simulink model "GA_tracking_sim"  (R2024a)
settings: Solver=FixedStepAuto  StartTime=0.0  StopTime=100  FixedStep=1e-3  RelTol=1e-3
InitFcn:
  | close;
  | % % z
  | k_p_z = -9.64;
  | k_i_z = -5.55;
  | k_d_z = -7.46;
  | k_a_z = 1.37;
  | %
  | % % psi
  | k_p_psi = 5.84;
  | k_d_psi = .836;
  | %
  | % % phi
  | k_p_phi = 2.33;
  | k_d_phi = 0.756;
  | %
  | % % tt
  | k_p_tt = 1;
  | k_d_tt = .302;
StopFcn:
  | % plot3(x,y,-z,['b','-'],x_g,y_g,z_g,['r','--'],'LineWidth',1.25);
  | % xlabel('x');
  | % ylabel('y');
  | % zlabel('z');
  | % grid on;
undefined symbols (not defined in the file or in its folder): k_a_phi, k_a_psi, k_a_tt, k_a_x, k_a_y, k_d_x, k_d_y, k_i_phi, k_i_psi, k_i_tt, k_i_x, k_i_y, k_p_x, k_p_y
libraries: simulink x6
settings Model: Creator=luand  LastModifiedBy=luand
settings DataIOCC: ReturnWorkspaceOutputs=off

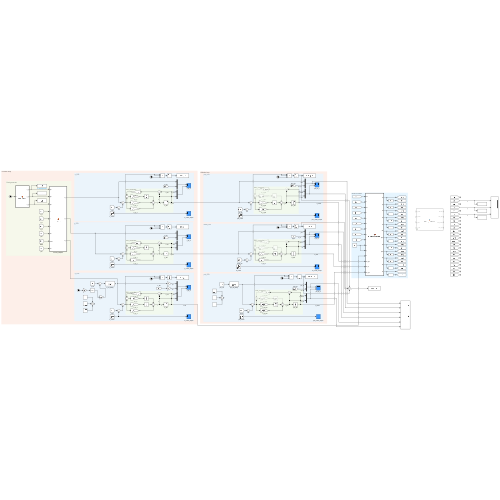
[thumbnail: Simulink's stored preview of the top-level diagram]
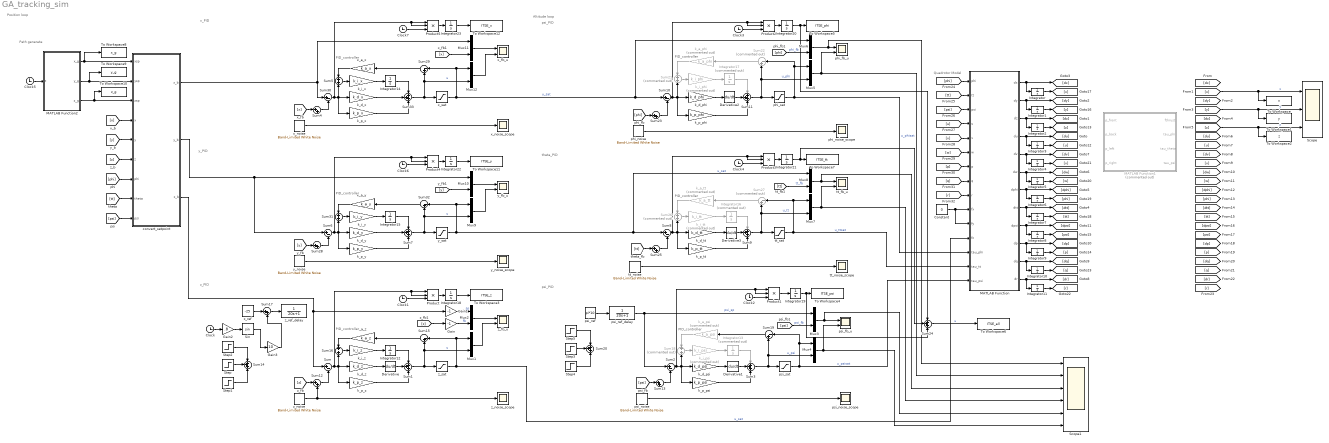
== system GA_tracking_sim ==
  note: Path generate
  note: Altitude loop
  note: z_PID
  note: PID_controller
  note: PID_controller
  note: psi_PID
  note: Quadrotor Model
  note: PID_controller
  note: PID_controller
  note: PID_controller
  note: PID_controller
  note: theta_PID
  note: psi_PID
  note: Position loop
  note: y_PID
  note: x_PID
  Clock{,1..7} (8 alike) : Clock
  Constant : Constant  Value=0
  Derivative{,1..3} (4 alike) : Derivative
  Gain : Gain  Gain=-1
  Gain1 : Gain  Gain=-1
  Gain2 : Gain  Gain=.8
  Gain3 : Gain  Gain=10
  Integrator : Integrator  UpperSaturationLimit=1000  LowerSaturationLimit=-1000
  Integrator1 : Integrator  UpperSaturationLimit=1000  LowerSaturationLimit=-1000
  Integrator{8..11} (4 alike) : Integrator  LimitOutput=on  UpperSaturationLimit=100  LowerSaturationLimit=-100
  Integrator12 : Integrator  UpperSaturationLimit=1000  LowerSaturationLimit=-1000
  Integrator13 : Integrator  Commented=on  LimitOutput=on  UpperSaturationLimit=1000  LowerSaturationLimit=-1000
  Integrator14 : Integrator
  Integrator15 : Integrator
  Integrator16 : Integrator  Commented=on
  Integrator17 : Integrator  Commented=on  LimitOutput=on  UpperSaturationLimit=1000  LowerSaturationLimit=-1000
  Integrator18 : Integrator  UpperSaturationLimit=100000  LowerSaturationLimit=-100000
  Integrator{19..23} (5 alike) : Integrator  LimitOutput=on  UpperSaturationLimit=100000  LowerSaturationLimit=-100000
  Integrator2 : Integrator  UpperSaturationLimit=0  LowerSaturationLimit=-1000
  Integrator3 : Integrator  LimitOutput=on  UpperSaturationLimit=10000  LowerSaturationLimit=-10000
  Integrator4 : Integrator  LimitOutput=on  UpperSaturationLimit=10000  LowerSaturationLimit=-10000
  Integrator5 : Integrator  LimitOutput=on  UpperSaturationLimit=10000  LowerSaturationLimit=-10000
  Integrator6 : Integrator  LimitOutput=on  UpperSaturationLimit=1000  LowerSaturationLimit=-1000
  Integrator7 : Integrator  LimitOutput=on  UpperSaturationLimit=1000  LowerSaturationLimit=-1000
  MATLAB Function : MATLAB Function  TreatAsAtomicUnit=on
  MATLAB Function1 : MATLAB Function  Commented=on  TreatAsAtomicUnit=on
  MATLAB Function2 : MATLAB Function  TreatAsAtomicUnit=on
  Mux{1..12} (12 alike) : Mux  Inputs=2
  Product{,1..5} (6 alike) : Product  Inputs=3
  Scope : Scope  NumInputPorts=3
  Scope1 : Scope  NumInputPorts=6
  Sin : Trigonometry
  Step : Step  Time=25  After=-20  SampleTime=0
  Step1 : Step  Time=40  After=15  SampleTime=0
  Step2 : Step  Time=10  After=-5  SampleTime=0
  Step3 : Step  Time=8  After=-6.28  SampleTime=0
  Step4 : Step  Time=17  After=6.28  SampleTime=0
  Step5 : Step  After=3.14  SampleTime=0
  Sum{,2,6,8,10,30} (6 alike) : Sum  Inputs=|+-
  Sum{1,3,7,9,11,14,20,24,33} (9 alike) : Sum  Inputs=+++
  Sum{4,12..13,17,23,25,28} (7 alike) : Sum  Inputs=|++
  Sum{15,19,29,32} (4 alike) : Sum  Inputs=|-+
  Sum16 : Sum  Inputs=+|+
  Sum18 : Sum  Commented=on  Inputs=+|+
  Sum21 : Sum  Commented=on  Inputs=+|+
  Sum22 : Sum  Commented=on  Inputs=|-+
  Sum26 : Sum  Commented=on  Inputs=+|+
  Sum27 : Sum  Commented=on  Inputs=|-+
  Sum31 : Sum  Inputs=+|+
  Sum5 : Sum  Inputs=+|+
  To Workspace : ToWorkspace  VariableName=x  SampleTime=-1
      settings: Save2DSignal=2-D array (concatenate along first dimension)
  To Workspace1 : ToWorkspace  VariableName=y  SampleTime=-1
      settings: Save2DSignal=2-D array (concatenate along first dimension)
  To Workspace10 : ToWorkspace  VariableName=z_g  SampleTime=-1
      settings: Save2DSignal=2-D array (concatenate along first dimension)
  To Workspace11 : ToWorkspace  VariableName=ITSE_y  SampleTime=-1
  To Workspace12 : ToWorkspace  VariableName=ITSE_x  SampleTime=-1
  To Workspace2 : ToWorkspace  VariableName=z  SampleTime=-1
      settings: Save2DSignal=2-D array (concatenate along first dimension)
  To Workspace3 : ToWorkspace  VariableName=ITSE_z  SampleTime=-1
  To Workspace4 : ToWorkspace  VariableName=ITSE_psi  SampleTime=-1
  To Workspace5 : ToWorkspace  VariableName=ITSE_phi  SampleTime=-1
  To Workspace6 : ToWorkspace  VariableName=ITSE_all  SampleTime=-1
  To Workspace7 : ToWorkspace  VariableName=ITSE_tt  SampleTime=-1
  To Workspace8 : ToWorkspace  VariableName=x_g  SampleTime=-1
      settings: Save2DSignal=2-D array (concatenate along first dimension)
  To Workspace9 : ToWorkspace  VariableName=y_g  SampleTime=-1
      settings: Save2DSignal=2-D array (concatenate along first dimension)
  convert_setpoint : MATLAB Function  TreatAsAtomicUnit=on
  k_a_phi : Gain  Commented=on  Gain=k_a_phi
  k_a_psi : Gain  Commented=on  Gain=k_a_psi
  k_a_tt : Gain  Commented=on  Gain=k_a_tt
  k_a_x : Gain  Gain=k_a_x
  k_a_y : Gain  Gain=k_a_y
  k_a_z : Gain  Gain=k_a_z
  k_d_phi : Gain  Gain=k_d_phi
  k_d_psi : Gain  Gain=k_d_psi
  k_d_tt : Gain  Gain=k_d_tt
  k_d_x : Gain  Gain=k_d_x
  k_d_y : Gain  Gain=k_d_y
  k_d_z : Gain  Gain=k_d_z
  k_i_phi : Gain  Commented=on  Gain=k_i_phi
  k_i_psi : Gain  Commented=on  Gain=k_i_psi
  k_i_tt : Gain  Commented=on  Gain=k_i_tt
  k_i_x : Gain  Gain=k_i_x
  k_i_y : Gain  Gain=k_i_y
  k_i_z : Gain  Gain=k_i_z
  k_p_phi : Gain  Gain=k_p_phi
  k_p_psi : Gain  Gain=k_p_psi
  k_p_tt : Gain  Gain=k_p_tt
  k_p_x : Gain  Gain=k_p_x
  k_p_y : Gain  Gain=k_p_y
  k_p_z : Gain  Gain=k_p_z
  phi_fb_u : Scope  NumInputPorts=2
  phi_noise : simulink/Sources/Band-Limited White Noise  Cov=[0.001]  Ts=0.1  seed=[23341]
  phi_noise_scope : Scope
  phi_sat : Saturate  UpperLimit=100  LowerLimit=-100
  psi_fb_u : Scope  NumInputPorts=2
  psi_noise : simulink/Sources/Band-Limited White Noise  Cov=[0.001]  Ts=0.1  seed=[23341]
  psi_noise_scope : Scope
  psi_ref : Constant  Value=pi*10
  psi_ref_delay : TransferFcn  Denominator=[20 1]
  psi_sat : Saturate  UpperLimit=50  LowerLimit=-50
  tt_fb_u : Scope  NumInputPorts=2
  tt_noise : simulink/Sources/Band-Limited White Noise  Cov=[0.001]  Ts=0.1  seed=[23341]
  tt_noise_scope : Scope
  tt_sat : Saturate  UpperLimit=100  LowerLimit=-100
  x_fb_u : Scope  NumInputPorts=2
  x_noise : simulink/Sources/Band-Limited White Noise  Cov=[0.01]  Ts=0.1  seed=[23341]
  x_noise_scope : Scope
  x_sat : Saturate  UpperLimit=pi/2  LowerLimit=-pi/2
  y_fb_u : Scope  NumInputPorts=2
  y_noise : simulink/Sources/Band-Limited White Noise  Cov=[0.01]  Ts=0.1  seed=[23341]
  y_noise_scope : Scope
  y_sat : Saturate  UpperLimit=pi/2  LowerLimit=-pi/2
  z_fb_u : Scope  NumInputPorts=2
  z_noise : simulink/Sources/Band-Limited White Noise  Cov=[0.01]  Ts=0.1  seed=[23341]
  z_noise_scope : Scope
  z_ref : Constant  Value=-25
  z_ref_delay : TransferFcn  Denominator=[20 1]
  z_sat : Saturate  UpperLimit=100  LowerLimit=0
  wires:
  z_ref/1 -> Sum17/1
  Gain3/1 -> Sum17/2
  Integrator18/1 -> To Workspace3/1
  k_a_phi/1 -> Sum21/1
  [phi] -> Sum23/1
  Sum23/1 -> Sum10/2
  Sum11/1 -> Mux5/2, Sum22/2, phi_sat/1  "u_phi"
  k_d_phi/1 -> Derivative2/1
  [phi] -> Mux6/2  "phi_fb"
  Mux5/1 -> phi_fb_u/2, Scope1/2
  Mux6/1 -> Scope1/1, phi_fb_u/1
  x_sat/1 -> Mux6/1, Sum10/1, Mux12/1, Sum29/1  "u_sat"
  Sum21/1 -> k_i_phi/1
  Clock1/1 -> Product/3
  [r] -> MATLAB Function/9(r)
  Step/1 -> Sum14/2
  Clock3/1 -> Product2/3
  psi_ref_delay/1 -> Sum2/1, Mux3/1  "psi_sp"
  phi_noise/1 -> phi_noise_scope/1
  Integrator8/1 -> [psi]
  Sum13/1 -> Sum2/2
  Sum19/1 -> k_a_psi/1
  Integrator19/1 -> Sum24/3, To Workspace4/1
  [psi] -> Mux3/2  "psi_fb"
  MATLAB Function/11(dq) -> Integrator10/1, [dq]
  Mux4/1 -> Scope1/6, psi_fb_u/2
  Constant/1 -> MATLAB Function/11(fy), MATLAB Function/10(fx)
  k_a_psi/1 -> Sum18/1
  Mux1/1 -> z_fb_u/2
  Mux3/1 -> psi_fb_u/1, Scope1/5
  Product1/1 -> Integrator19/1
  Step5/1 -> Sum20/1
  Step4/1 -> Sum20/3
  k_p_psi/1 -> Sum3/3
  Derivative1/1 -> Sum3/2
  Gain/1 -> Mux2/2  "fb"
  Integrator5/1 -> [w]
  [tt] -> MATLAB Function/2(tt)
  Sum22/1 -> k_a_phi/1
  k_p_phi/1 -> Sum11/3
  [x] -> Scope/1, To Workspace/1  "x"
  Integrator/1 -> [x]
  psi_sat/1 -> Sum19/1, Mux4/1, MATLAB Function/15(tau_psi)  "u_psisat"
  MATLAB Function/4(du) -> Integrator3/1, [du]
  k_d_psi/1 -> Derivative1/1
  Sin/1 -> Gain3/1
  Sum16/1 -> k_i_z/1
  Integrator12/1 -> Sum1/1
  k_a_z/1 -> Sum16/1
  Mux2/1 -> z_fb_u/1
  Gain1/1 -> Mux2/1  "sp"
  Step1/1 -> Sum14/3
  [phi] -> MATLAB Function/1(phi)
  k_d_z/1 -> Derivative/1
  Product/1 -> Integrator18/1
  Clock/1 -> Gain2/1
  z_noise/1 -> Sum12/2, z_noise_scope/1
  Gain2/1 -> Sin/1
  Integrator10/1 -> [q]
  k_i_z/1 -> Integrator12/1
  [y] -> Scope/2, To Workspace1/1  "y"
  Sum1/1 -> Sum15/2, Mux1/2, z_sat/1  "u"
  Step2/1 -> Sum14/1
  [psi] -> Sum13/1
  Sum18/1 -> k_i_psi/1
  Derivative2/1 -> Sum11/2
  [psi] -> MATLAB Function/3(psi)
  k_i_phi/1 -> Integrator17/1
  Derivative/1 -> Sum1/2
  Clock2/1 -> Product1/3
  phi_sat/1 -> Mux5/1, Sum22/1, MATLAB Function/13(tau_phi)  "u_phisat"
  k_p_z/1 -> Sum1/3
  k_i_tt/1 -> Integrator16/1
  k_i_y/1 -> Integrator15/1
  Product2/1 -> Integrator20/1
  z_sat/1 -> Mux1/1, Sum15/1, MATLAB Function/12(fz)  "u_sat"
  Step3/1 -> Sum20/2
  [p] -> MATLAB Function/7(p)
  MATLAB Function/1(dx) -> Integrator/1, [dx]
  Integrator7/1 -> [tt]
  Sum2/1 -> Product1/1, Product1/2, Sum18/2, k_d_psi/1, k_p_psi/1
  Integrator20/1 -> Sum24/1, To Workspace5/1
  Integrator1/1 -> [y]
  Sum12/1 -> Sum/2
  Sum/1 -> Product/1, Product/2, k_d_z/1, k_p_z/1, Sum16/2
  [z] -> Scope/3, To Workspace2/1  "z"
  MATLAB Function/2(dy) -> Integrator1/1, [dy]
  k_i_psi/1 -> Integrator13/1
  Integrator3/1 -> [u]
  Sum3/1 -> psi_sat/1, Mux4/2, Sum19/2  "u_psi"
  Integrator2/1 -> [z]
  [w] -> MATLAB Function/6(w)
  Integrator11/1 -> [r]
  Integrator9/1 -> [p]
  [u] -> MATLAB Function/4(u)
  Integrator6/1 -> [phi]
  MATLAB Function/5(dv) -> Integrator4/1, [dv]
  psi_noise/1 -> psi_noise_scope/1
  MATLAB Function/6(dw) -> Integrator5/1, [dw]
  [z] -> Gain/1
  Integrator4/1 -> [v]
  MATLAB Function/12(dr) -> Integrator11/1, [dr]
  MATLAB Function/9(dpsi) -> Integrator8/1, [dpsi]
  [q] -> MATLAB Function/8(q)
  Sum10/1 -> k_d_phi/1, Sum21/2, k_p_phi/1, Product2/2, Product2/1
  [v] -> MATLAB Function/5(v)
  [z] -> Sum12/1
  MATLAB Function/10(dp) -> Integrator9/1, [dp]
  MATLAB Function/8(dtt) -> Integrator7/1, [dtt]
  Sum15/1 -> k_a_z/1
  MATLAB Function/3(dz) -> Integrator2/1, [dz]
  MATLAB Function/7(dphi) -> Integrator6/1, [dphi]
  Integrator17/1 -> Sum11/1
  Sum17/1 -> z_ref_delay/1
  psi_ref/1 -> psi_ref_delay/1
  Sum24/1 -> To Workspace6/1  "u"
  [tt] -> Sum25/1
  Sum25/1 -> Sum8/2
  Integrator16/1 -> Sum9/1
  k_p_tt/1 -> Sum9/3
  Sum26/1 -> k_i_tt/1
  k_d_tt/1 -> Derivative3/1
  Derivative3/1 -> Sum9/2
  k_a_tt/1 -> Sum26/1
  Sum27/1 -> k_a_tt/1
  tt_sat/1 -> Mux7/1, Sum27/1, MATLAB Function/14(tau_tt)  "u_ttsat"
  y_sat/1 -> Mux8/1, Sum8/1, Mux9/1, Sum32/1  "u_sat"
  Mux8/1 -> tt_fb_u/1, Scope1/3
  Mux7/1 -> Scope1/4, tt_fb_u/2
  [tt] -> Mux8/2  "tt_fb"
  Sum9/1 -> Mux7/2, Sum27/2, tt_sat/1  "u_tt"
  tt_noise/1 -> tt_noise_scope/1
  Sum8/1 -> k_d_tt/1, Sum26/2, k_p_tt/1, Product3/1, Product3/2
  Integrator21/1 -> Sum24/2, To Workspace7/1
  Product3/1 -> Integrator21/1
  Integrator13/1 -> Sum3/1
  Clock4/1 -> Product3/3
  Clock5/1 -> MATLAB Function2/1(t)
  MATLAB Function2/2(y_g) -> To Workspace9/1, convert_setpoint/2(ysp)
  MATLAB Function2/1(x_g) -> convert_setpoint/1(xsp), To Workspace8/1
  MATLAB Function2/3(z_g) -> To Workspace10/1, convert_setpoint/3(zsp)
  [x] -> convert_setpoint/4(x)
  [y] -> convert_setpoint/5(y)
  [z] -> convert_setpoint/6(z)
  [phi] -> convert_setpoint/7(phi)
  [tt] -> convert_setpoint/8(theta)
  [psi] -> convert_setpoint/9(psi)
  k_d_y/1 -> Sum7/2
  Integrator15/1 -> Sum7/1
  k_p_y/1 -> Sum7/3
  Sum31/1 -> k_i_y/1
  k_a_y/1 -> Sum31/1
  Sum7/1 -> Mux9/2, Sum32/2, y_sat/1  "u"
  Sum32/1 -> k_a_y/1
  [y] -> Sum28/1
  y_noise/1 -> y_noise_scope/1
  Sum6/1 -> k_d_y/1, k_p_y/1, Sum31/2, Product4/2, Product4/1
  Product4/1 -> Integrator22/1
  Clock6/1 -> Product4/3
  Integrator22/1 -> To Workspace11/1
  Integrator23/1 -> To Workspace12/1
  Clock7/1 -> Product5/3
  Product5/1 -> Integrator23/1
  Sum30/1 -> Product5/1, Product5/2, Sum5/2, k_p_x/1, k_d_x/1
  x_noise/1 -> x_noise_scope/1
  [x] -> Sum4/1
  Sum29/1 -> k_a_x/1
  Sum33/1 -> x_sat/1, Sum29/2, Mux12/2  "u"
  k_a_x/1 -> Sum5/1
  Sum5/1 -> k_i_x/1
  k_p_x/1 -> Sum33/3
  Integrator14/1 -> Sum33/1
  k_d_x/1 -> Sum33/2
  k_i_x/1 -> Integrator14/1
  convert_setpoint/1(x_b) -> Sum30/1, Mux11/1
  convert_setpoint/2(y_b) -> Sum6/1, Mux10/1
  Sum28/1 -> Sum6/2
  [y] -> Mux10/2
  Mux10/1 -> y_fb_u/1
  Mux9/1 -> y_fb_u/2
  Mux11/1 -> x_fb_u/1
  Mux12/1 -> x_fb_u/2
  Sum4/1 -> Sum30/2
  [x] -> Mux11/2
  convert_setpoint/3(z_b) -> Sum/1, Gain1/1

== matlab function GA_tracking_sim/MATLAB Function1 ==
  data: fthrust output; tau_phi output; tau_theta output; tau_psi output; p_front input; p_back input; p_left input; p_right input
function [fthrust, tau_phi, tau_theta, tau_psi] = Motor_dynamics(p_front, p_back, p_left, p_right)

fthrust = k_thrust*(p_front+p_back+p_left+p_right);
tau_phi = l*k_thrust*(-p_right+p_left);
tau_theta = l*k_thrust*(p_front+p_back);
tau_psi = k_momen*(-p_front-p_back+p_left+p_right);

== matlab function GA_tracking_sim/MATLAB Function ==
  data: phi input; tt input; psi input; u input; dx output; v input; w input; p input; q input; r input; fx input; fy input; fz input; tau_phi input; tau_tt input; tau_psi input; dy output; dz output; du output; dv output; dw output; dphi output; dtt output; dpsi output; dp output; dq output; dr output
function [dx,dy,dz,du,dv,dw,dphi,dtt,dpsi,dp,dq,dr]=Dynamics_plustype(phi,tt,psi,u,v,w,p,q,r,fx,fy,fz,tau_phi,tau_tt,tau_psi)

% Eqs. 16-19

M = .75;
m = .05;
g = 9.81;
R = .03;
l = .22;

Jx = .4*M*R*R+2*l*l*m;
Jy = .4*M*R*R+2*l*l*m;
Jz = .4*M*R*R+4*l*l*m;

dx = cos(tt)*cos(psi)*u+(sin(phi)*sin(tt)*cos(psi)-cos(phi)*sin(psi))*v+(cos(phi)*sin(tt)*cos(psi)+sin(phi)*sin(psi))*w;
dy = cos(tt)*sin(psi)*u+(sin(phi)*sin(tt)*sin(psi)+cos(phi)*cos(psi))*v+(cos(phi)*sin(tt)*sin(psi)-sin(phi)*cos(psi))*w;
dz = -(sin(tt)*u-sin(phi)*cos(tt)*v-cos(phi)*cos(tt)*w);

du = (r*v-q*w)-g*sin(tt);
dv = (p*w-r*u)+g*cos(tt)*sin(phi);
dw = (q*u-p*v)+g*cos(tt)*cos(phi)-fz/(M+4*m);

dphi = p+sin(phi)*tan(phi)*q+cos(phi)*tan(tt)*r;
dtt  = cos(phi)*q-sin(phi)*r;
dpsi = sin(phi)*q/cos(tt)+cos(phi)*r/cos(tt);

dp = ((Jy-Jz)*q*r+tau_phi)/Jx;
dq = ((Jz-Jx)*p*r+tau_tt)/Jy;
dr = ((Jx-Jy)*q*p+tau_psi)/Jz;

== matlab function GA_tracking_sim/MATLAB Function2 ==
  data: t input; x_g output; y_g output; z_g output
function [x_g,y_g,z_g] = path_ground(t)

A = 5; % x range
a = 5; % grid x
B = 5; % y range
b = 4; % grid y
C = 10;% z range 
coef = .07;
x_g = A*cos(a*coef*t);
y_g = B*sin(b*coef*t);
z_g = -C*(1-exp(-5*coef*t));

== matlab function GA_tracking_sim/convert_setpoint ==
  data: xsp input; x_b output; y_b output; ysp input; zsp input; x input; y input; z input; phi input; theta input; psi input; z_b output
function [x_b,y_b,z_b] = convert_setpoint(xsp,ysp,zsp,x,y,z,phi,theta,psi)
xyz_sp_g = [xsp ysp zsp 1];

R_body_to_ground = [cos(psi)*cos(theta) cos(psi)*sin(theta)*sin(phi)-sin(psi)*cos(phi) cos(psi)*sin(theta)*cos(phi)+sin(psi)*sin(phi);
                    sin(psi)*cos(theta) sin(psi)*sin(theta)*sin(phi)+cos(psi)*cos(phi) sin(psi)*sin(theta)*cos(phi)-cos(psi)*sin(phi);
                    -sin(theta) cos(theta)*sin(phi) cos(theta)*cos(phi)];
P_body_to_ground = [x y z]';
% T_body_to_ground = [R_body_to_ground P_body_to_ground; 0 0 0 1];

P_ground_to_body = [-P_body_to_ground'*R_body_to_ground(:,1);
                    -P_body_to_ground'*R_body_to_ground(:,2);
                    -P_body_to_ground'*R_body_to_ground(:,3)];
T_ground_to_body = [R_body_to_ground' P_ground_to_body; 0 0 0 1];

xyz_sp_b = T_ground_to_body*xyz_sp_g';

x_b = xyz_sp_b(1);
y_b = xyz_sp_b(2);
Z_b = xyz_sp_b(3);
